simulink model "valores_de_entrada"  (R2019a)
settings: Solver=VariableStepAuto  StartTime=0.0  StopTime=10.0  RelTol=1e-3
settings Model: Creator=hecto  LastModifiedBy=hecto

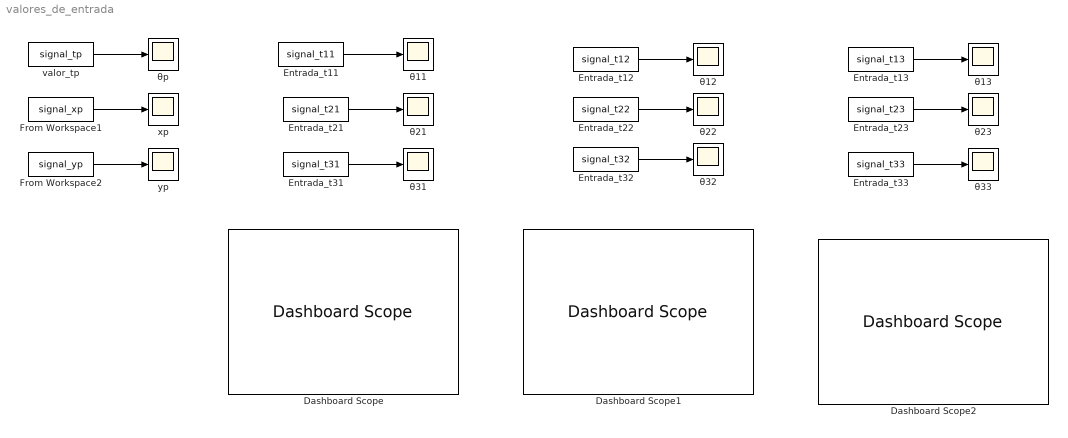
== system valores_de_entrada ==
  Dashboard Scope : DashboardScope
  Dashboard Scope1 : DashboardScope
  Dashboard Scope2 : DashboardScope
  Entrada_t11 : FromWorkspace  VariableName=signal_t11  SampleTime=0
  Entrada_t12 : FromWorkspace  VariableName=signal_t12  SampleTime=0
  Entrada_t13 : FromWorkspace  VariableName=signal_t13  SampleTime=0
  Entrada_t21 : FromWorkspace  VariableName=signal_t21  SampleTime=0
  Entrada_t22 : FromWorkspace  VariableName=signal_t22  SampleTime=0
  Entrada_t23 : FromWorkspace  VariableName=signal_t23  SampleTime=0
  Entrada_t31 : FromWorkspace  VariableName=signal_t31  SampleTime=0
  Entrada_t32 : FromWorkspace  VariableName=signal_t32  SampleTime=0
  Entrada_t33 : FromWorkspace  VariableName=signal_t33  SampleTime=0
  From Workspace1 : FromWorkspace  VariableName=signal_xp  SampleTime=0
  From Workspace2 : FromWorkspace  VariableName=signal_yp  SampleTime=0
  "valor_tp " : FromWorkspace  VariableName=signal_tp  SampleTime=0
  xp : Scope
  yp : Scope
  θ{11..13,21..23,31..33} (9 alike) : Scope
  θp : Scope
  wires:
  From Workspace2/1 -> yp/1
  From Workspace1/1 -> xp/1
  "valor_tp "/1 -> θp/1
  Entrada_t11/1 -> θ11/1
  Entrada_t12/1 -> θ12/1
  Entrada_t21/1 -> θ21/1
  Entrada_t22/1 -> θ22/1
  Entrada_t23/1 -> θ23/1
  Entrada_t13/1 -> θ13/1
  Entrada_t31/1 -> θ31/1
  Entrada_t32/1 -> θ32/1
  Entrada_t33/1 -> θ33/1
